simulink subsystem "DCMotorModel"  (R2023b)
settings: Solver=VariableStepAuto  StartTime=0.0  StopTime=10.0  RelTol=1e-3
values from neighbouring files (symbols this model uses):
  c = 20    [main.m]
  gear_ratio = 3    [main.m]
  La = 0.15*10^-3    (= 0.00015)    [main.m]
  Ra = 0.035    [main.m]
undefined symbols (not defined in the file or in its folder): J, K_B, K_T
settings Model: Creator=Bronz  LastModifiedBy=kai
settings ModelReferenceCC: EnableRefExpFcnMdlSchedulingChecks=on

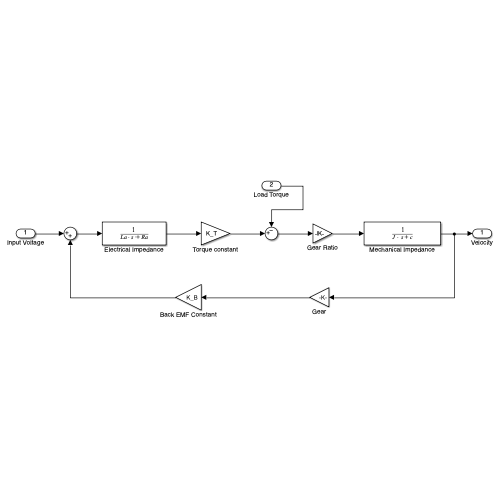
[thumbnail: Simulink's stored preview of the top-level diagram]
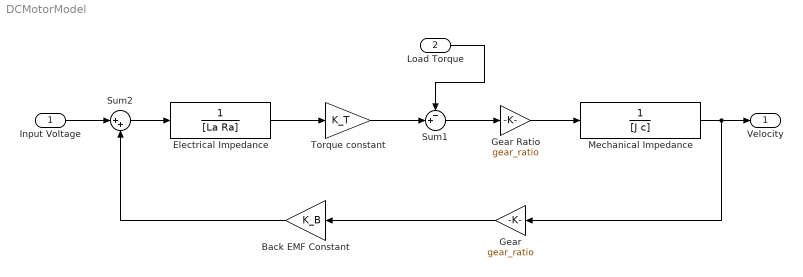
== system DCMotorModel ==
  Input Voltage : Inport
  Load Torque : Inport  Port=2
  Back EMF Constant : Gain  Gain=K_B  ParamDataTypeStr=Inherit: Inherit from 'Gain'
  Electrical Impedance : TransferFcn  Denominator=[La Ra]
  Gear : Gain  Gain=gear_ratio  ParamDataTypeStr=Inherit: Inherit from 'Gain'
  Gear Ratio : Gain  Gain=gear_ratio
  Mechanical Impedance : TransferFcn  Denominator=[J c]
  Sum1 : Sum  Inputs=-+|
  Sum2 : Sum  Inputs=|++
  Torque constant : Gain  Gain=K_T
  Velocity : Outport
  wires:
  Electrical Impedance/1 -> Torque constant/1
  Input Voltage/1 -> Sum2/1
  Sum2/1 -> Electrical Impedance/1
  Mechanical Impedance/1 -> Gear/1, Velocity/1
  Back EMF Constant/1 -> Sum2/2
  Torque constant/1 -> Sum1/2
  Load Torque/1 -> Sum1/1
  Sum1/1 -> Gear Ratio/1
  Gear Ratio/1 -> Mechanical Impedance/1
  Gear/1 -> Back EMF Constant/1
